simulink model "modelo_planta"  (R2023b)
settings: Solver=VariableStepAuto  StartTime=0.0  StopTime=10.0  RelTol=1e-3
settings Model: Creator=Nahuel  LastModifiedBy=Nahuel

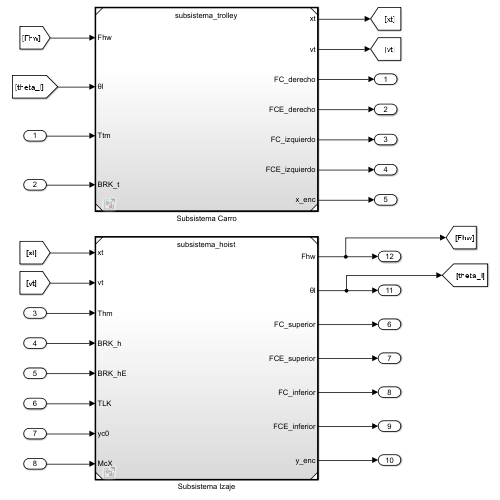
[thumbnail: Simulink's stored preview of the top-level diagram]
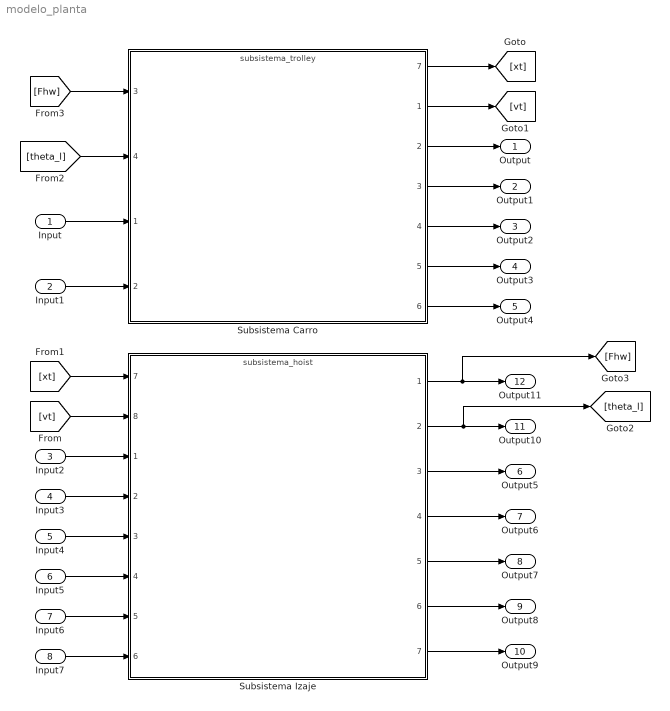
== system modelo_planta ==
  Input : Inport
  Input1 : Inport  Port=2
  Input2 : Inport  Port=3
  Input3 : Inport  Port=4
  Input4 : Inport  Port=5
  Input5 : Inport  Port=6
  Input6 : Inport  Port=7
  Input7 : Inport  Port=8
  Subsistema Carro : ModelReference  ModelNameDialog=subsistema_trolley.slx  SimulationMode=Normal  ModelReferenceVersion=1.32
      settings: PortSchema="{\"entries\":[{\"content\":{\"sides\":[{\"content\":{\"connectorIds\":[\"In3\",\"In4\",\"In1\",\"In2\"]},\"type\":\"ConnectorPlacement.EquallySpacedRectSide\",\"uuid\":\"36720be2-f819-438f-b04c-00f8672fc6a8\"},{\"content\":{\"connectorIds\":[\"Out7\",\"Out1\",\"Out2\",\"Out3\",\"Out4\",\"Out5\",\"Out6\"],\"side\":\"RIGHT\"},\"type\":\"ConnectorPlacement.EquallySpacedRectSide\",\"uuid\":\"552285d0-0ffb-402a-9325-fd99e08cb345\"},{\"content\":{\"side\":\"TOP\"},\"type\":\"ConnectorPlacement.EquallySpacedRectSide\",\"uuid\":\"94baa680-e0a6-40c3-ba7d-6a7aba77d5b5\"}]},\"type\":\"ConnectorPlacement.EquallySpacedConnector\",\"uuid\":\"4dc8347a-6d40-4f6d-a2bc-9f8e2d1ea62c\"}],\"packageUris\":[\"http://schema.mathworks.com/mf0/Connector/R2020b\"],\"version\":\"1.0\"}"
  Subsistema Izaje : ModelReference  ModelNameDialog=subsistema_hoist.slx  SimulationMode=Normal  ModelReferenceVersion=1.40
      settings: PortSchema="{\"entries\":[{\"content\":{\"sides\":[{\"content\":{\"connectorIds\":[\"In7\",\"In8\",\"In1\",\"In2\",\"In3\",\"In4\",\"In5\",\"In6\"]},\"type\":\"ConnectorPlacement.EquallySpacedRectSide\",\"uuid\":\"349e0789-ef5a-4031-9c4b-8690978ba87e\"},{\"content\":{\"connectorIds\":[\"Out1\",\"Out2\",\"Out3\",\"Out4\",\"Out5\",\"Out6\",\"Out7\"],\"side\":\"RIGHT\"},\"type\":\"ConnectorPlacement.EquallySpacedRectSide\",\"uuid\":\"7f933b24-aef9-4898-9c3b-c3a037c44f97\"},{\"content\":{\"side\":\"TOP\"},\"type\":\"ConnectorPlacement.EquallySpacedRectSide\",\"uuid\":\"8171a877-1b67-48a2-b648-b4955358868b\"}]},\"type\":\"ConnectorPlacement.EquallySpacedConnector\",\"uuid\":\"ee1f183e-c091-4662-bb61-234d7a2aecd5\"}],\"packageUris\":[\"http://schema.mathworks.com/mf0/Connector/R2020b\"],\"version\":\"1.0\"}"
  Output : Outport
  Output1 : Outport  Port=2
  Output2 : Outport  Port=3
  Output3 : Outport  Port=4
  Output4 : Outport  Port=5
  Output5 : Outport  Port=6
  Output6 : Outport  Port=7
  Output7 : Outport  Port=8
  Output8 : Outport  Port=9
  Output9 : Outport  Port=10
  Output10 : Outport  Port=11
  Output11 : Outport  Port=12
  wires:
  [vt] -> Subsistema Izaje/8
  [xt] -> Subsistema Izaje/7
  Subsistema Izaje/2 -> Output10/1, [theta_l]
  [theta_l] -> Subsistema Carro/4
  Subsistema Izaje/1 -> [Fhw], Output11/1
  [Fhw] -> Subsistema Carro/3
  Subsistema Carro/7 -> [xt]
  Subsistema Carro/1 -> [vt]
  Input/1 -> Subsistema Carro/1
  Input1/1 -> Subsistema Carro/2
  Input2/1 -> Subsistema Izaje/1
  Input3/1 -> Subsistema Izaje/2
  Input4/1 -> Subsistema Izaje/3
  Input5/1 -> Subsistema Izaje/4
  Input6/1 -> Subsistema Izaje/5
  Input7/1 -> Subsistema Izaje/6
  Subsistema Carro/2 -> Output/1
  Subsistema Carro/5 -> Output3/1
  Subsistema Carro/4 -> Output2/1
  Subsistema Carro/3 -> Output1/1
  Subsistema Carro/6 -> Output4/1
  Subsistema Izaje/3 -> Output5/1
  Subsistema Izaje/4 -> Output6/1
  Subsistema Izaje/5 -> Output7/1
  Subsistema Izaje/6 -> Output8/1
  Subsistema Izaje/7 -> Output9/1
